simulink model "platoon_project_string_stability3"  (Simulink 8.9)
settings: Solver=FixedStepAuto  StartTime=0.0  StopTime=80  FixedStep=0.02  RelTol=1e-3  EnableMultiTasking=on
model workspace (MAT data in the model file):
  Kd_brake = 1
  Kd_throttle = 500
  Ki_brake = 1
  Ki_throttle = 120
  Kp_brake = 8000
  Kp_throttle = 50
  L = 15
  V0 = 21
  k1 = 0.001
  k2 = -1.004
  q = 0.2
  tau : num (value not decoded)
undefined symbols (not defined in the file): c_aero, delay_brake, F_roll, h, I_e, I_wheel, KB, mass, max_throttle, max_throttle_rate, min_throttle, mu_B, mu_C, mu_D, mu_E, P_po, Rdrive, sigbuilder_block, tau_brake, tau_throttle, throttle_o, tnet_table, w_wheel_o, we_max, we_min, we_o, x_dot_o
libraries: simulink x6
(part 1 of 2)
settings Model: Creator=user  LastModifiedBy=edward
settings SolverCC: AutoInsertRateTranBlk=on
settings DataIOCC: SaveOutput=off  SaveTime=off
settings OptimizationCC: DefaultParameterBehavior=Inlined  InlineInvariantSignals=on  PassReuseOutputArgsAs=Individual arguments  ExpressionDepthLimit=2147483647  StateBitsets=on  DataBitsets=on  ZeroExternalMemoryAtStartup=off  ZeroInternalMemoryAtStartup=off  NoFixptDivByZeroProtection=on  LifeSpan=1
settings DebuggingCC: SolverPrmCheckMsg=warning  ParameterTunabilityLossMsg=error  FcnCallInpInsideContextMsg=error
settings HardwareCC: ProdIntDivRoundTo=Floor  ProdEndianess=LittleEndian  ProdHWDeviceType=Generic->Custom
settings SFSimCC: MATLABDynamicMemAlloc=off
settings RTWCC: SystemTargetFile=ert.tlc  TLCOptions=-p0  GenCodeOnly=on  TemplateMakefile=ert_default_tmf  Description=Embedded Coder  GenerateReport=on  RTWVerbose=off  IncludeHyperlinkInReport=on  LaunchReport=on  GenerateTraceInfo=on  GenerateTraceReport=on  GenerateTraceReportSl=on  GenerateTraceReportSf=on  GenerateTraceReportEml=on
settings CodeAppCC: ForceParamTrailComments=on  IgnoreCustomStorageClasses=off  OperatorAnnotations=on  SimulinkDataObjDesc=on  SFDataObjDesc=on  MATLABFcnDesc=on  CustomSymbolStrGlobalVar=rt$N$M  CustomSymbolStrType=$N$M  CustomSymbolStrFcn=$N$M$F  CustomSymbolStrMacro=$N$M  InsertBlockDesc=on  MATLABSourceComments=on
settings ERTTargetCC: CodeReplacementLibrary=ISO_C  GenerateSampleERTMain=on  IncludeMdlTerminateFcn=off  SuppressErrorStatus=on  SupportAbsoluteTime=off  SupportNonFinite=off  SupportComplex=off  PurelyIntegerCode=on  InlinedParameterPlacement=NonHierarchical  RootIOFormat=Structure reference  ERTCustomFileTemplate=example_file_process.tlc

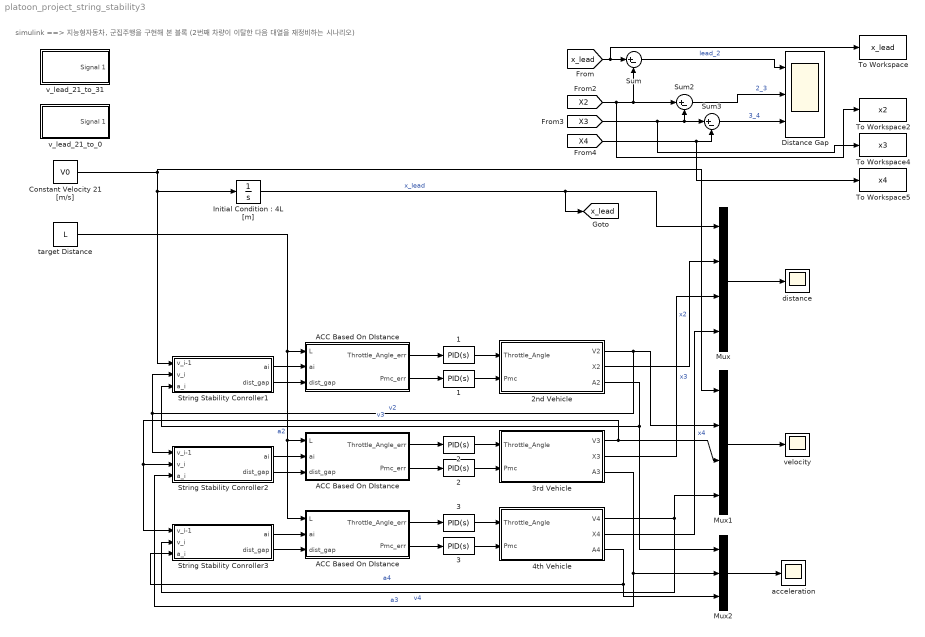
== system platoon_project_string_stability3 ==
  note: simulink ==> 지능형자동차, 군집주행을 구현해 본 블록 (2번째 차량이 이탈한 다음 대열을 재정비하는 시나리오)
  "               ACC Based On DIstance            " : MATLAB Function  TreatAsAtomicUnit=on
  "               ACC Based On DIstance             " : MATLAB Function  TreatAsAtomicUnit=on
  "               ACC Based On DIstance              " : MATLAB Function  TreatAsAtomicUnit=on
  "  1" : simulink/Continuous/PID Controller  Controller=PID  TimeDomain=Continuous-time  SampleTime=-1  IntegratorMethod=Forward Euler  FilterMethod=Forward Euler  Form=Parallel  UseFilter=on  ControllerParametersSource=internal  P=Kp_brake  I=Ki_brake  D=Kd_brake  N=100  InitialConditionSource=internal  InitialConditionForIntegrator=0  InitialConditionForFilter=0  ExternalReset=none  LimitOutput=off  UpperSaturationLimit=inf  LowerSaturationLimit=-inf  LinearizeAsGain=on  AntiWindupMode=none  Kb=1  TrackingMode=off  Kt=1  PParamMin=[]  PParamMax=[]  IParamMin=[]  IParamMax=[]  DParamMin=[]  DParamMax=[]  NParamMin=[]  NParamMax=[]  KbParamMin=[]  KbParamMax=[]  KtParamMin=[]  KtParamMax=[]  POutMin=[]  POutMax=[]  IOutMin=[]  IOutMax=[]  DOutMin=[]  DOutMax=[]  NOutMin=[]  NOutMax=[]  KbOutMin=[]  KbOutMax=[]  KtOutMin=[]  KtOutMax=[]  IntegratorOutMin=[]  IntegratorOutMax=[]  FilterOutMin=[]  FilterOutMax=[]  SumOutMin=[]  SumOutMax=[]  SumI1OutMin=[]  SumI1OutMax=[]  SumI2OutMin=[]  SumI2OutMax=[]  SumI3OutMin=[]  SumI3OutMax=[]  SumDOutMin=[]  SumDOutMax=[]  SaturationOutMin=[]  SaturationOutMax=[]  IntegratorContinuousStateAttributes=''  IntegratorStateMustResolveToSignalObject=off  IntegratorRTWStateStorageClass=Auto  FilterContinuousStateAttributes=''  FilterStateMustResolveToSignalObject=off  FilterRTWStateStorageClass=Auto  DifferentiatorICPrevScaledInput=0  DifferentiatorOutMin=[]  DifferentiatorOutMax=[]  InitialConditionSetting=State (most efficient)
  "  2" : simulink/Continuous/PID Controller  Controller=PID  TimeDomain=Continuous-time  SampleTime=-1  IntegratorMethod=Forward Euler  FilterMethod=Forward Euler  Form=Parallel  UseFilter=on  ControllerParametersSource=internal  P=Kp_brake  I=Ki_brake  D=Kd_brake  N=100  InitialConditionSource=internal  InitialConditionForIntegrator=0  InitialConditionForFilter=0  ExternalReset=none  LimitOutput=off  UpperSaturationLimit=inf  LowerSaturationLimit=-inf  LinearizeAsGain=on  AntiWindupMode=none  Kb=1  TrackingMode=off  Kt=1  PParamMin=[]  PParamMax=[]  IParamMin=[]  IParamMax=[]  DParamMin=[]  DParamMax=[]  NParamMin=[]  NParamMax=[]  KbParamMin=[]  KbParamMax=[]  KtParamMin=[]  KtParamMax=[]  POutMin=[]  POutMax=[]  IOutMin=[]  IOutMax=[]  DOutMin=[]  DOutMax=[]  NOutMin=[]  NOutMax=[]  KbOutMin=[]  KbOutMax=[]  KtOutMin=[]  KtOutMax=[]  IntegratorOutMin=[]  IntegratorOutMax=[]  FilterOutMin=[]  FilterOutMax=[]  SumOutMin=[]  SumOutMax=[]  SumI1OutMin=[]  SumI1OutMax=[]  SumI2OutMin=[]  SumI2OutMax=[]  SumI3OutMin=[]  SumI3OutMax=[]  SumDOutMin=[]  SumDOutMax=[]  SaturationOutMin=[]  SaturationOutMax=[]  IntegratorContinuousStateAttributes=''  IntegratorStateMustResolveToSignalObject=off  IntegratorRTWStateStorageClass=Auto  FilterContinuousStateAttributes=''  FilterStateMustResolveToSignalObject=off  FilterRTWStateStorageClass=Auto  DifferentiatorICPrevScaledInput=0  DifferentiatorOutMin=[]  DifferentiatorOutMax=[]  InitialConditionSetting=State (most efficient)
  "  3" : simulink/Continuous/PID Controller  Controller=PID  TimeDomain=Continuous-time  SampleTime=-1  IntegratorMethod=Forward Euler  FilterMethod=Forward Euler  Form=Parallel  UseFilter=on  ControllerParametersSource=internal  P=Kp_brake  I=Ki_brake  D=Kd_brake  N=100  InitialConditionSource=internal  InitialConditionForIntegrator=0  InitialConditionForFilter=0  ExternalReset=none  LimitOutput=off  UpperSaturationLimit=inf  LowerSaturationLimit=-inf  LinearizeAsGain=on  AntiWindupMode=none  Kb=1  TrackingMode=off  Kt=1  PParamMin=[]  PParamMax=[]  IParamMin=[]  IParamMax=[]  DParamMin=[]  DParamMax=[]  NParamMin=[]  NParamMax=[]  KbParamMin=[]  KbParamMax=[]  KtParamMin=[]  KtParamMax=[]  POutMin=[]  POutMax=[]  IOutMin=[]  IOutMax=[]  DOutMin=[]  DOutMax=[]  NOutMin=[]  NOutMax=[]  KbOutMin=[]  KbOutMax=[]  KtOutMin=[]  KtOutMax=[]  IntegratorOutMin=[]  IntegratorOutMax=[]  FilterOutMin=[]  FilterOutMax=[]  SumOutMin=[]  SumOutMax=[]  SumI1OutMin=[]  SumI1OutMax=[]  SumI2OutMin=[]  SumI2OutMax=[]  SumI3OutMin=[]  SumI3OutMax=[]  SumDOutMin=[]  SumDOutMax=[]  SaturationOutMin=[]  SaturationOutMax=[]  IntegratorContinuousStateAttributes=''  IntegratorStateMustResolveToSignalObject=off  IntegratorRTWStateStorageClass=Auto  FilterContinuousStateAttributes=''  FilterStateMustResolveToSignalObject=off  FilterRTWStateStorageClass=Auto  DifferentiatorICPrevScaledInput=0  DifferentiatorOutMin=[]  DifferentiatorOutMax=[]  InitialConditionSetting=State (most efficient)
  " 1" : simulink/Continuous/PID Controller  Controller=PID  TimeDomain=Continuous-time  SampleTime=-1  IntegratorMethod=Forward Euler  FilterMethod=Forward Euler  Form=Parallel  UseFilter=on  ControllerParametersSource=internal  P=Kp_throttle  I=Ki_throttle  D=Kd_throttle  N=100  InitialConditionSource=internal  InitialConditionForIntegrator=0  InitialConditionForFilter=0  ExternalReset=none  LimitOutput=off  UpperSaturationLimit=inf  LowerSaturationLimit=-inf  LinearizeAsGain=on  AntiWindupMode=none  Kb=1  TrackingMode=off  Kt=1  PParamMin=[]  PParamMax=[]  IParamMin=[]  IParamMax=[]  DParamMin=[]  DParamMax=[]  NParamMin=[]  NParamMax=[]  KbParamMin=[]  KbParamMax=[]  KtParamMin=[]  KtParamMax=[]  POutMin=[]  POutMax=[]  IOutMin=[]  IOutMax=[]  DOutMin=[]  DOutMax=[]  NOutMin=[]  NOutMax=[]  KbOutMin=[]  KbOutMax=[]  KtOutMin=[]  KtOutMax=[]  IntegratorOutMin=[]  IntegratorOutMax=[]  FilterOutMin=[]  FilterOutMax=[]  SumOutMin=[]  SumOutMax=[]  SumI1OutMin=[]  SumI1OutMax=[]  SumI2OutMin=[]  SumI2OutMax=[]  SumI3OutMin=[]  SumI3OutMax=[]  SumDOutMin=[]  SumDOutMax=[]  SaturationOutMin=[]  SaturationOutMax=[]  IntegratorContinuousStateAttributes=''  IntegratorStateMustResolveToSignalObject=off  IntegratorRTWStateStorageClass=Auto  FilterContinuousStateAttributes=''  FilterStateMustResolveToSignalObject=off  FilterRTWStateStorageClass=Auto  DifferentiatorICPrevScaledInput=0  DifferentiatorOutMin=[]  DifferentiatorOutMax=[]  InitialConditionSetting=State (most efficient)
  " 2" : simulink/Continuous/PID Controller  Controller=PID  TimeDomain=Continuous-time  SampleTime=-1  IntegratorMethod=Forward Euler  FilterMethod=Forward Euler  Form=Parallel  UseFilter=on  ControllerParametersSource=internal  P=Kp_throttle  I=Ki_throttle  D=Kd_throttle  N=100  InitialConditionSource=internal  InitialConditionForIntegrator=0  InitialConditionForFilter=0  ExternalReset=none  LimitOutput=off  UpperSaturationLimit=inf  LowerSaturationLimit=-inf  LinearizeAsGain=on  AntiWindupMode=none  Kb=1  TrackingMode=off  Kt=1  PParamMin=[]  PParamMax=[]  IParamMin=[]  IParamMax=[]  DParamMin=[]  DParamMax=[]  NParamMin=[]  NParamMax=[]  KbParamMin=[]  KbParamMax=[]  KtParamMin=[]  KtParamMax=[]  POutMin=[]  POutMax=[]  IOutMin=[]  IOutMax=[]  DOutMin=[]  DOutMax=[]  NOutMin=[]  NOutMax=[]  KbOutMin=[]  KbOutMax=[]  KtOutMin=[]  KtOutMax=[]  IntegratorOutMin=[]  IntegratorOutMax=[]  FilterOutMin=[]  FilterOutMax=[]  SumOutMin=[]  SumOutMax=[]  SumI1OutMin=[]  SumI1OutMax=[]  SumI2OutMin=[]  SumI2OutMax=[]  SumI3OutMin=[]  SumI3OutMax=[]  SumDOutMin=[]  SumDOutMax=[]  SaturationOutMin=[]  SaturationOutMax=[]  IntegratorContinuousStateAttributes=''  IntegratorStateMustResolveToSignalObject=off  IntegratorRTWStateStorageClass=Auto  FilterContinuousStateAttributes=''  FilterStateMustResolveToSignalObject=off  FilterRTWStateStorageClass=Auto  DifferentiatorICPrevScaledInput=0  DifferentiatorOutMin=[]  DifferentiatorOutMax=[]  InitialConditionSetting=State (most efficient)
  " 3" : simulink/Continuous/PID Controller  Controller=PID  TimeDomain=Continuous-time  SampleTime=-1  IntegratorMethod=Forward Euler  FilterMethod=Forward Euler  Form=Parallel  UseFilter=on  ControllerParametersSource=internal  P=Kp_throttle  I=Ki_throttle  D=Kd_throttle  N=100  InitialConditionSource=internal  InitialConditionForIntegrator=0  InitialConditionForFilter=0  ExternalReset=none  LimitOutput=off  UpperSaturationLimit=inf  LowerSaturationLimit=-inf  LinearizeAsGain=on  AntiWindupMode=none  Kb=1  TrackingMode=off  Kt=1  PParamMin=[]  PParamMax=[]  IParamMin=[]  IParamMax=[]  DParamMin=[]  DParamMax=[]  NParamMin=[]  NParamMax=[]  KbParamMin=[]  KbParamMax=[]  KtParamMin=[]  KtParamMax=[]  POutMin=[]  POutMax=[]  IOutMin=[]  IOutMax=[]  DOutMin=[]  DOutMax=[]  NOutMin=[]  NOutMax=[]  KbOutMin=[]  KbOutMax=[]  KtOutMin=[]  KtOutMax=[]  IntegratorOutMin=[]  IntegratorOutMax=[]  FilterOutMin=[]  FilterOutMax=[]  SumOutMin=[]  SumOutMax=[]  SumI1OutMin=[]  SumI1OutMax=[]  SumI2OutMin=[]  SumI2OutMax=[]  SumI3OutMin=[]  SumI3OutMax=[]  SumDOutMin=[]  SumDOutMax=[]  SaturationOutMin=[]  SaturationOutMax=[]  IntegratorContinuousStateAttributes=''  IntegratorStateMustResolveToSignalObject=off  IntegratorRTWStateStorageClass=Auto  FilterContinuousStateAttributes=''  FilterStateMustResolveToSignalObject=off  FilterRTWStateStorageClass=Auto  DifferentiatorICPrevScaledInput=0  DifferentiatorOutMin=[]  DifferentiatorOutMax=[]  InitialConditionSetting=State (most efficient)
  2nd Vehicle : Subsystem
  3rd Vehicle : Subsystem
  4th Vehicle : Subsystem
  Constant Velocity 21 [m/s] : Constant  Value=V0
  Distance Gap : Scope  NumInputPorts=3
  "Initial Condition : 4L [m]" : Integrator  InitialCondition=4*L
  Mux : Mux
  Mux1 : Mux
  Mux2 : Mux  Inputs=3
  String Stability Conroller1 : Subsystem
  String Stability Conroller2 : Subsystem
  String Stability Conroller3 : Subsystem
  Sum : Sum  Inputs=|+-
  Sum2 : Sum  Inputs=|+-
  Sum3 : Sum  Inputs=|+-
  To Workspace : ToWorkspace  VariableName=x_lead  SampleTime=-1
  To Workspace2 : ToWorkspace  VariableName=x2  SampleTime=-1
  To Workspace4 : ToWorkspace  VariableName=x3  SampleTime=-1
  To Workspace5 : ToWorkspace  VariableName=x4  SampleTime=-1
  acceleration : Scope
  distance : Scope
  target Distance : Constant  Value=L
  v_lead_21_to_0 : Subsystem  Tag=STV Subsys  LoadFcn=sigbuilder_block('load');  StartFcn=sigbuilder_block('start');  StopFcn=sigbuilder_block('stop');  ClipboardFcn=sigbuilder_block('clipboard');  mask(Sigbuilder block){tuvar=[0:10]}
      mask help: Simulink:masks:SigbuilderBlock_MD
      mask init:
      | if ~strcmp(get_param(bdroot(gcbh),'SimulationStatus'),'stopped') tuvar = sigbuilder_block('maskInit'); end
      settings: CopyFcn=sigbuilder_block('copy');  DeleteFcn=sigbuilder_block('delete');  ModelCloseFcn=sigbuilder_block('modelClose');  PreSaveFcn=sigbuilder_block('preSave');  PauseFcn=sigbuilder_block('pause');  ContinueFcn=sigbuilder_block('continue');  NameChangeFcn=sigbuilder_block('namechange');  OpenFcn=sigbuilder_block('open',[434.4 168 550.8 400.2 ]);  CloseFcn=sigbuilder_block('close');
      mask Display: plot(0, 0, 100, 100,[2, 2, 32, 32, 2], [68, 8, 8, 68, 68],[32, 2], [38, 38], [32, 19, 2],[53, 60, 44], [32, 17, 17, 2],[16, 16, 31, 31]);txt = getActiveGroup(gcbh);text(2, 100, txt,'verticalAlignment', 'top');
  v_lead_21_to_31 : Subsystem  Tag=STV Subsys  LoadFcn=sigbuilder_block('load');  StartFcn=sigbuilder_block('start');  StopFcn=sigbuilder_block('stop');  ClipboardFcn=sigbuilder_block('clipboard');  mask(Sigbuilder block){tuvar=[0:10]}
      mask help: Simulink:masks:SigbuilderBlock_MD
      mask init:
      | if ~strcmp(get_param(bdroot(gcbh),'SimulationStatus'),'stopped') tuvar = sigbuilder_block('maskInit'); end
      settings: CopyFcn=sigbuilder_block('copy');  DeleteFcn=sigbuilder_block('delete');  ModelCloseFcn=sigbuilder_block('modelClose');  PreSaveFcn=sigbuilder_block('preSave');  PauseFcn=sigbuilder_block('pause');  ContinueFcn=sigbuilder_block('continue');  NameChangeFcn=sigbuilder_block('namechange');  OpenFcn=sigbuilder_block('open',[434.4 168 550.8 400.2 ]);  CloseFcn=sigbuilder_block('close');
      mask Display: plot(0, 0, 100, 100,[2, 2, 32, 32, 2], [68, 8, 8, 68, 68],[32, 2], [38, 38], [32, 19, 2],[53, 60, 44], [32, 17, 17, 2],[16, 16, 31, 31]);txt = getActiveGroup(gcbh);text(2, 100, txt,'verticalAlignment', 'top');
  velocity : Scope
  tag scope: x_lead=global
  wires:
  "Initial Condition : 4L [m]"/1 -> Mux/1, [x_lead]  "x_lead"
  " 1"/1 -> 2nd Vehicle/1(Throttle_Angle)
  "  1"/1 -> 2nd Vehicle/2(Pmc)
  Mux/1 -> distance/1
  String Stability Conroller1/1(ai) -> "               ACC Based On DIstance            "/2(ai)
  "               ACC Based On DIstance            "/2(Pmc_err) -> "  1"/1
  "               ACC Based On DIstance            "/1(Throttle_Angle_err) -> " 1"/1
  2nd Vehicle/1(V2) -> Mux1/2, String Stability Conroller2/1(v_i-1), String Stability Conroller1/2(v_i)  "v2"
  2nd Vehicle/3(A2) -> Mux2/1, String Stability Conroller1/3(a_i)  "a2"
  2nd Vehicle/2(X2) -> Mux/2  "x2"
  Mux2/1 -> acceleration/1
  "               ACC Based On DIstance              "/1(Throttle_Angle_err) -> " 2"/1
  "               ACC Based On DIstance              "/2(Pmc_err) -> "  2"/1
  String Stability Conroller2/1(ai) -> "               ACC Based On DIstance              "/2(ai)
  String Stability Conroller3/1(ai) -> "               ACC Based On DIstance             "/2(ai)
  "               ACC Based On DIstance             "/2(Pmc_err) -> "  3"/1
  "               ACC Based On DIstance             "/1(Throttle_Angle_err) -> " 3"/1
  " 2"/1 -> 3rd Vehicle/1(Throttle_Angle)
  "  2"/1 -> 3rd Vehicle/2(Pmc)
  " 3"/1 -> 4th Vehicle/1(Throttle_Angle)
  "  3"/1 -> 4th Vehicle/2(Pmc)
  3rd Vehicle/1(V3) -> Mux1/3, String Stability Conroller3/1(v_i-1), String Stability Conroller2/2(v_i)  "v3"
  3rd Vehicle/3(A3) -> Mux2/2, String Stability Conroller2/3(a_i)  "a3"
  3rd Vehicle/2(X3) -> Mux/3  "x3"
  4th Vehicle/2(X4) -> Mux/4  "x4"
  4th Vehicle/1(V4) -> Mux1/4, String Stability Conroller3/2(v_i)  "v4"
  4th Vehicle/3(A4) -> Mux2/3, String Stability Conroller3/3(a_i)  "a4"
  Constant Velocity 21 [m/s]/1 -> Mux1/1, String Stability Conroller1/1(v_i-1), "Initial Condition : 4L [m]"/1
  [x_lead] -> To Workspace/1, Sum/1
  [X3] -> To Workspace4/1, Sum3/1, Sum2/2
  [X4] -> To Workspace5/1, Sum3/2
  Sum/1 -> Distance Gap/1  "lead_2"
  Sum2/1 -> Distance Gap/2  "2_3"
  Sum3/1 -> Distance Gap/3  "3_4"
  String Stability Conroller1/2(dist_gap) -> "               ACC Based On DIstance            "/3(dist_gap)
  String Stability Conroller2/2(dist_gap) -> "               ACC Based On DIstance              "/3(dist_gap)
  String Stability Conroller3/2(dist_gap) -> "               ACC Based On DIstance             "/3(dist_gap)
  [X2] -> To Workspace2/1, Sum/2, Sum2/1
  target Distance/1 -> "               ACC Based On DIstance             "/1(L), "               ACC Based On DIstance              "/1(L), "               ACC Based On DIstance            "/1(L)
  Mux1/1 -> velocity/1

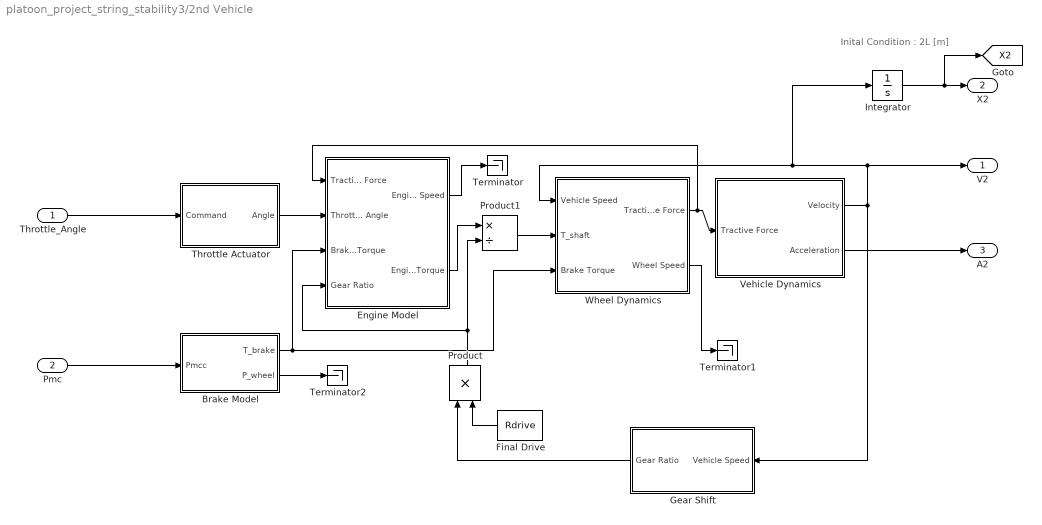
== system platoon_project_string_stability3/2nd Vehicle ==
  note: Inital Condition : 2L [m]
  Throttle_Angle : Inport
  Pmc : Inport  Port=2
  Brake Model : Subsystem
  Engine Model : Subsystem
  Final Drive : Constant  Value=Rdrive
  Gear Shift : Subsystem
  Integrator : Integrator  InitialCondition=2*L
  Product : Product  Inputs=**  SaturateOnIntegerOverflow=on  RndMeth=Zero  InputSameDT=on  OutDataTypeStr=Inherit: Same as first input
  Product1 : Product  Inputs=*/  SaturateOnIntegerOverflow=on  RndMeth=Zero  InputSameDT=on  OutDataTypeStr=Inherit: Same as first input
  Terminator : Terminator
  Terminator1 : Terminator
  Terminator2 : Terminator
  Throttle Actuator : Subsystem
  Vehicle Dynamics : Subsystem
  Wheel Dynamics : Subsystem
  V2 : Outport
  X2 : Outport  Port=2
  A2 : Outport  Port=3
  tag scope: X2=global
  wires:
  Integrator/1 -> [X2], X2/1
  Vehicle Dynamics/2(Acceleration) -> A2/1
  Brake Model/2(P_wheel) -> Terminator2/1
  Wheel Dynamics/2(Wheel Speed) -> Terminator1/1
  Engine Model/1(Engine Speed) -> Terminator/1
  Product1/1 -> Wheel Dynamics/2(T_shaft)
  Engine Model/2(Engine Torque) -> Product1/1
  Brake Model/1(T_brake) -> Engine Model/3(Brake Torque), Wheel Dynamics/3(Brake Torque)
  Product/1 -> Product1/2, Engine Model/4(Gear Ratio)
  Final Drive/1 -> Product/2
  Gear Shift/1(Gear Ratio) -> Product/1
  Wheel Dynamics/1(Tractive Force) -> Vehicle Dynamics/1(Tractive Force), Engine Model/1(Tractive Force)
  Throttle Actuator/1(Angle) -> Engine Model/2(Throttle Angle)
  Throttle_Angle/1 -> Throttle Actuator/1(Command)
  Pmc/1 -> Brake Model/1(Pmcc)
  Vehicle Dynamics/1(Velocity) -> Wheel Dynamics/1(Vehicle Speed), Integrator/1, V2/1, Gear Shift/1(Vehicle Speed)

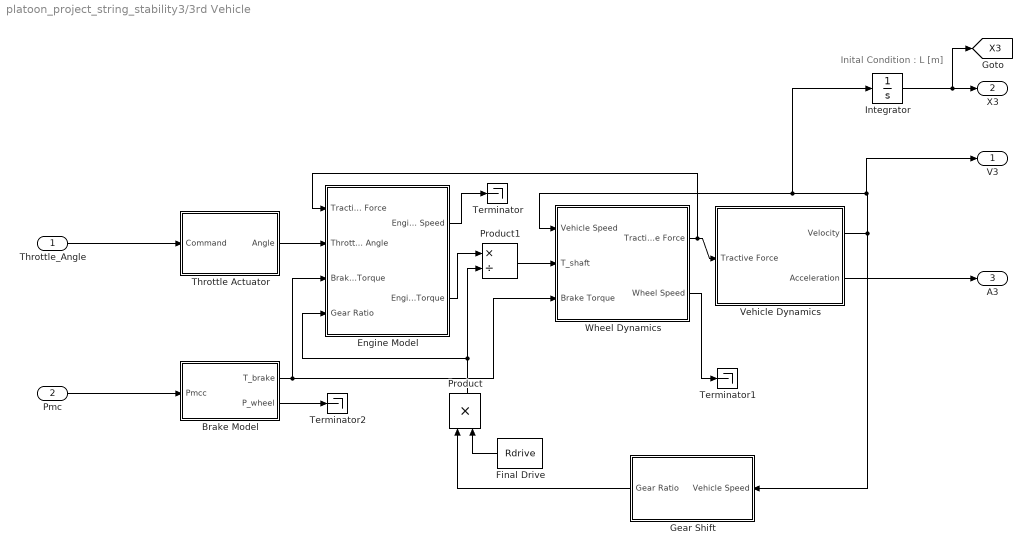
== system platoon_project_string_stability3/3rd Vehicle ==
  note: Inital Condition : L [m]
  Throttle_Angle : Inport
  Pmc : Inport  Port=2
  Brake Model : Subsystem
  Engine Model : Subsystem
  Final Drive : Constant  Value=Rdrive
  Gear Shift : Subsystem
  Integrator : Integrator  InitialCondition=L
  Product : Product  Inputs=**  SaturateOnIntegerOverflow=on  RndMeth=Zero  InputSameDT=on  OutDataTypeStr=Inherit: Same as first input
  Product1 : Product  Inputs=*/  SaturateOnIntegerOverflow=on  RndMeth=Zero  InputSameDT=on  OutDataTypeStr=Inherit: Same as first input
  Terminator : Terminator
  Terminator1 : Terminator
  Terminator2 : Terminator
  Throttle Actuator : Subsystem
  Vehicle Dynamics : Subsystem
  Wheel Dynamics : Subsystem
  V3 : Outport
  X3 : Outport  Port=2
  A3 : Outport  Port=3
  tag scope: X3=global
  wires:
  Pmc/1 -> Brake Model/1(Pmcc)
  Throttle_Angle/1 -> Throttle Actuator/1(Command)
  Throttle Actuator/1(Angle) -> Engine Model/2(Throttle Angle)
  Wheel Dynamics/1(Tractive Force) -> Engine Model/1(Tractive Force), Vehicle Dynamics/1(Tractive Force)
  Gear Shift/1(Gear Ratio) -> Product/1
  Final Drive/1 -> Product/2
  Product/1 -> Engine Model/4(Gear Ratio), Product1/2
  Brake Model/1(T_brake) -> Wheel Dynamics/3(Brake Torque), Engine Model/3(Brake Torque)
  Engine Model/2(Engine Torque) -> Product1/1
  Product1/1 -> Wheel Dynamics/2(T_shaft)
  Engine Model/1(Engine Speed) -> Terminator/1
  Wheel Dynamics/2(Wheel Speed) -> Terminator1/1
  Brake Model/2(P_wheel) -> Terminator2/1
  Vehicle Dynamics/2(Acceleration) -> A3/1
  Vehicle Dynamics/1(Velocity) -> Gear Shift/1(Vehicle Speed), V3/1, Integrator/1, Wheel Dynamics/1(Vehicle Speed)
  Integrator/1 -> [X3], X3/1

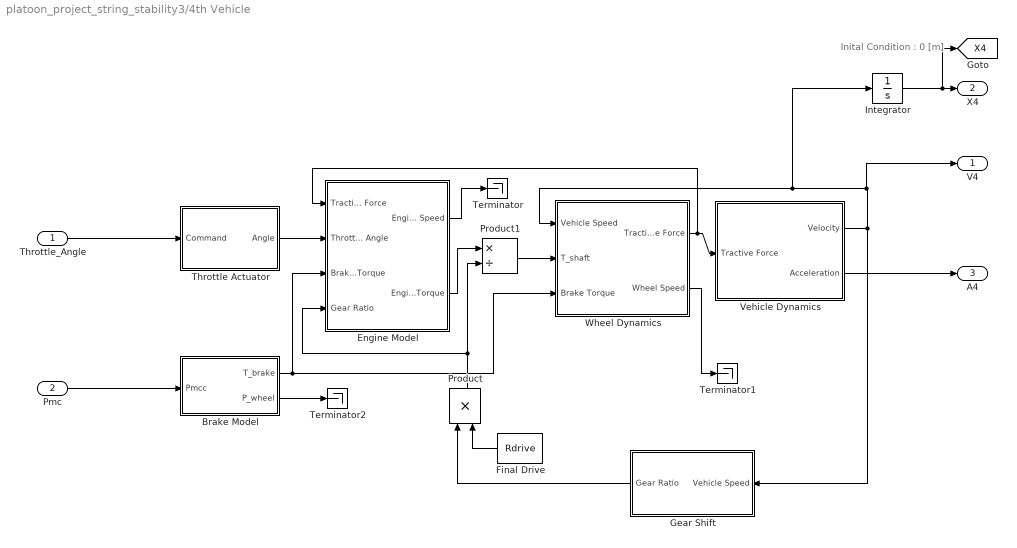
== system platoon_project_string_stability3/4th Vehicle ==
  note: Inital Condition : 0 [m]
  Throttle_Angle : Inport
  Pmc : Inport  Port=2
  Brake Model : Subsystem
  Engine Model : Subsystem
  Final Drive : Constant  Value=Rdrive
  Gear Shift : Subsystem
  Integrator : Integrator
  Product : Product  Inputs=**  SaturateOnIntegerOverflow=on  RndMeth=Zero  InputSameDT=on  OutDataTypeStr=Inherit: Same as first input
  Product1 : Product  Inputs=*/  SaturateOnIntegerOverflow=on  RndMeth=Zero  InputSameDT=on  OutDataTypeStr=Inherit: Same as first input
  Terminator : Terminator
  Terminator1 : Terminator
  Terminator2 : Terminator
  Throttle Actuator : Subsystem
  Vehicle Dynamics : Subsystem
  Wheel Dynamics : Subsystem
  V4 : Outport
  X4 : Outport  Port=2
  A4 : Outport  Port=3
  tag scope: X4=global
  wires:
  Integrator/1 -> [X4], X4/1
  Vehicle Dynamics/2(Acceleration) -> A4/1
  Brake Model/2(P_wheel) -> Terminator2/1
  Wheel Dynamics/2(Wheel Speed) -> Terminator1/1
  Engine Model/1(Engine Speed) -> Terminator/1
  Product1/1 -> Wheel Dynamics/2(T_shaft)
  Engine Model/2(Engine Torque) -> Product1/1
  Brake Model/1(T_brake) -> Engine Model/3(Brake Torque), Wheel Dynamics/3(Brake Torque)
  Product/1 -> Product1/2, Engine Model/4(Gear Ratio)
  Final Drive/1 -> Product/2
  Gear Shift/1(Gear Ratio) -> Product/1
  Wheel Dynamics/1(Tractive Force) -> Vehicle Dynamics/1(Tractive Force), Engine Model/1(Tractive Force)
  Throttle Actuator/1(Angle) -> Engine Model/2(Throttle Angle)
  Throttle_Angle/1 -> Throttle Actuator/1(Command)
  Pmc/1 -> Brake Model/1(Pmcc)
  Vehicle Dynamics/1(Velocity) -> V4/1, Wheel Dynamics/1(Vehicle Speed), Integrator/1, Gear Shift/1(Vehicle Speed)

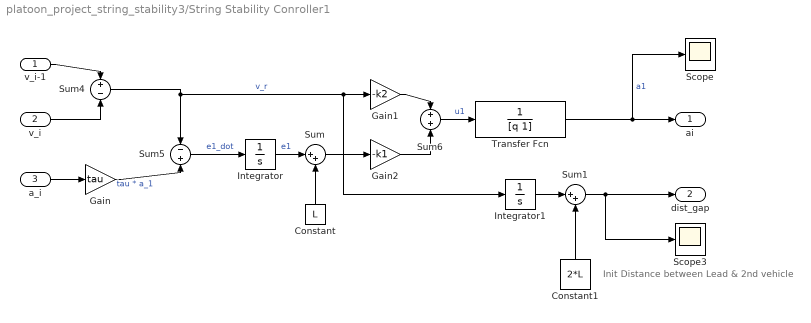
== system platoon_project_string_stability3/String Stability Conroller1 ==
  note: Init Distance between Lead & 2nd vehicle
  v_i-1 : Inport
  v_i : Inport  Port=2
  a_i : Inport  Port=3
  Constant : Constant  Value=L
  Constant1 : Constant  Value=2*L
  Gain : Gain  Gain=tau
  Gain1 : Gain  Gain=-k2
  Gain2 : Gain  Gain=-k1
  Integrator : Integrator
  Integrator1 : Integrator
  Scope : Scope
  Scope3 : Scope
  Sum : Sum  Inputs=|++
  Sum1 : Sum  Inputs=|++
  Sum4 : Sum  Inputs=+|-
  Sum5 : Sum  Inputs=-|+
  Sum6 : Sum  Inputs=+|+
  Transfer Fcn : TransferFcn  Denominator=[q 1]
  ai : Outport
  dist_gap : Outport  Port=2
  wires:
  v_i-1/1 -> Sum4/1
  v_i/1 -> Sum4/2
  a_i/1 -> Gain/1
  Sum6/1 -> Transfer Fcn/1  "u1"
  Gain/1 -> Sum5/2  "tau * a_1"
  Sum5/1 -> Integrator/1  "e1_dot"
  Gain2/1 -> Sum6/2
  Gain1/1 -> Sum6/1
  Transfer Fcn/1 -> Scope/1, ai/1  "a1"
  Constant/1 -> Sum/2
  Sum/1 -> Gain2/1
  Integrator/1 -> Sum/1  "e1"
  Sum4/1 -> Integrator1/1, Gain1/1, Sum5/1  "v_r"
  Integrator1/1 -> Sum1/1
  Sum1/1 -> dist_gap/1, Scope3/1
  Constant1/1 -> Sum1/2

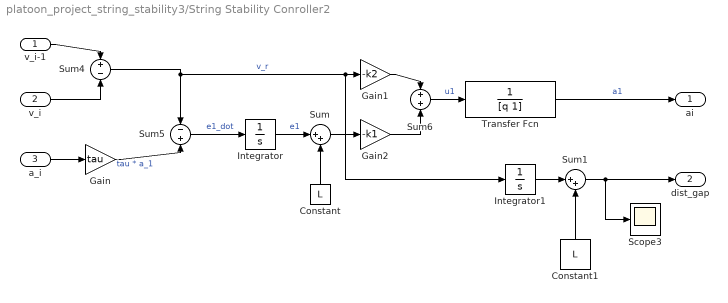
== system platoon_project_string_stability3/String Stability Conroller2 ==
  v_i-1 : Inport
  v_i : Inport  Port=2
  a_i : Inport  Port=3
  Constant : Constant  Value=L
  Constant1 : Constant  Value=L
  Gain : Gain  Gain=tau
  Gain1 : Gain  Gain=-k2
  Gain2 : Gain  Gain=-k1
  Integrator : Integrator
  Integrator1 : Integrator
  Scope3 : Scope
  Sum : Sum  Inputs=|++
  Sum1 : Sum  Inputs=|++
  Sum4 : Sum  Inputs=+|-
  Sum5 : Sum  Inputs=-|+
  Sum6 : Sum  Inputs=+|+
  Transfer Fcn : TransferFcn  Denominator=[q 1]
  ai : Outport
  dist_gap : Outport  Port=2
  wires:
  Gain1/1 -> Sum6/1
  Gain2/1 -> Sum6/2
  Sum5/1 -> Integrator/1  "e1_dot"
  Gain/1 -> Sum5/2  "tau * a_1"
  Sum6/1 -> Transfer Fcn/1  "u1"
  Transfer Fcn/1 -> ai/1  "a1"
  a_i/1 -> Gain/1
  v_i/1 -> Sum4/2
  v_i-1/1 -> Sum4/1
  Constant/1 -> Sum/2
  Sum/1 -> Gain2/1
  Integrator/1 -> Sum/1  "e1"
  Sum4/1 -> Sum5/1, Integrator1/1, Gain1/1  "v_r"
  Integrator1/1 -> Sum1/1
  Sum1/1 -> dist_gap/1, Scope3/1
  Constant1/1 -> Sum1/2

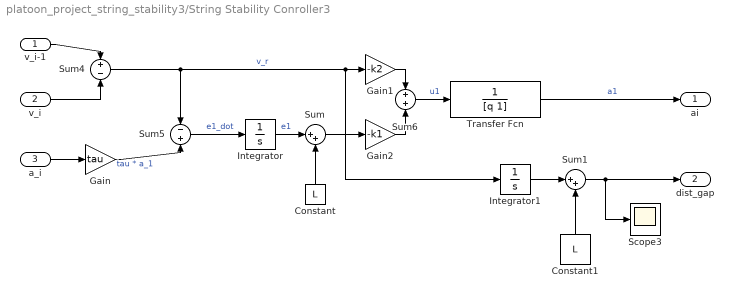
== system platoon_project_string_stability3/String Stability Conroller3 ==
  v_i-1 : Inport
  v_i : Inport  Port=2
  a_i : Inport  Port=3
  Constant : Constant  Value=L
  Constant1 : Constant  Value=L
  Gain : Gain  Gain=tau
  Gain1 : Gain  Gain=-k2
  Gain2 : Gain  Gain=-k1
  Integrator : Integrator
  Integrator1 : Integrator
  Scope3 : Scope
  Sum : Sum  Inputs=|++
  Sum1 : Sum  Inputs=|++
  Sum4 : Sum  Inputs=+|-
  Sum5 : Sum  Inputs=-|+
  Sum6 : Sum  Inputs=+|+
  Transfer Fcn : TransferFcn  Denominator=[q 1]
  ai : Outport
  dist_gap : Outport  Port=2
  wires:
  v_i-1/1 -> Sum4/1
  v_i/1 -> Sum4/2
  a_i/1 -> Gain/1
  Transfer Fcn/1 -> ai/1  "a1"
  Sum6/1 -> Transfer Fcn/1  "u1"
  Gain/1 -> Sum5/2  "tau * a_1"
  Sum5/1 -> Integrator/1  "e1_dot"
  Gain2/1 -> Sum6/2
  Gain1/1 -> Sum6/1
  Constant/1 -> Sum/2
  Sum/1 -> Gain2/1
  Integrator/1 -> Sum/1  "e1"
  Sum4/1 -> Sum5/1, Integrator1/1, Gain1/1  "v_r"
  Integrator1/1 -> Sum1/1
  Sum1/1 -> dist_gap/1, Scope3/1
  Constant1/1 -> Sum1/2

== system platoon_project_string_stability3/v_lead_21_to_0 ==
  Demux : Demux  Tag=STV Demux  Outputs=1
  FromWs : FromWorkspace  Tag=STV FromWs  VariableName=tuvar  SampleTime=0  SigBuilderData=DataTag1  VnvData=DataTag2
      SigBuilderData=|
      | common.afterFinalStr = 'Extrapolate'
      | common.sampleTime = 0
      | dataSet.timeRange = [0 20]
      | dataSet.name = 'Senario 2'
      | sbobj.Groups.Name = 'Senario 2'
      | sbobj.Groups.Signals.Name = 'Signal 1'
      | sbobj.Groups.Signals.XData = [0 5 8 20]
      | sbobj.Groups.Signals.YData = [21 21 5 5]
      | sbobj.Groups.TimeRange = [0 20]
  Signal 1 : Outport  Tag=STV Outport
  wires:
  Demux/1 -> Signal 1/1
  FromWs/1 -> Demux/1

== system platoon_project_string_stability3/v_lead_21_to_31 ==
  Demux : Demux  Tag=STV Demux  Outputs=1
  FromWs : FromWorkspace  Tag=STV FromWs  VariableName=tuvar  SampleTime=0  SigBuilderData=DataTag3  VnvData=DataTag4
      SigBuilderData=|
      | common.afterFinalStr = 'Extrapolate'
      | common.sampleTime = 0
      | dataSet.timeRange = [0 20]
      | dataSet.name = 'Senario 1'
      | sbobj.Groups.Name = 'Senario 1'
      | sbobj.Groups.Signals.Name = 'Signal 1'
      | sbobj.Groups.Signals.XData = [0 5 8 20]
      | sbobj.Groups.Signals.YData = [21 21 31 31]
      | sbobj.Groups.TimeRange = [0 20]
  Signal 1 : Outport  Tag=STV Outport
  wires:
  FromWs/1 -> Demux/1
  Demux/1 -> Signal 1/1

== system platoon_project_string_stability3/2nd Vehicle/Brake Model ==
  note: Wheel Pressure가 브레이크 패드에 있는
      | Spring(k)보다 크게 걸렸을 때에만 브레이크가 작동하므로
      | Dead Zone이 발생한다
  note: Wheel pressure
  note: brake는 1차 전달함수의 response를 보인다
  note: Valve를 여닫는 시간에 따라
      | 필연적으로 발생하는 Time Delay
  Pmcc : Inport
  Brake Coefficient : Gain  Gain=KB  SaturateOnIntegerOverflow=on  OutDataTypeStr=Inherit: Same as input  ParamDataTypeStr=Inherit: Same as input
  Brake Dynamics : TransferFcn  Denominator=[tau_brake 1]
  Dead Zone : DeadZone  LowerValue=-P_po  UpperValue=P_po  SaturateOnIntegerOverflow=on
  Pure Time Delay : TransportDelay  DelayTime=delay_brake
  T_brake : Outport
  P_wheel : Outport  Port=2
  wires:
  Brake Coefficient/1 -> T_brake/1
  Dead Zone/1 -> Brake Coefficient/1
  Brake Dynamics/1 -> P_wheel/1, Dead Zone/1  "P_wheel"
  Pmcc/1 -> Pure Time Delay/1
  Pure Time Delay/1 -> Brake Dynamics/1

== system platoon_project_string_stability3/2nd Vehicle/Engine Model ==
  note: engine map이 저장되어있다
      | 2-D Lookup table
      |
      | input : Throttle angle, Engine speed
      | output : Engine torque
  Tractive Force : Inport
  Throttle Angle : Inport  Port=2
  Brake Torque : Inport  Port=3
  Gear Ratio : Inport  Port=4
  1/(I_e+4*I_w*R^2) : Fcn  Expr=u(1)/(I_e+4*I_wheel*u(2)^2)
  Integrator : Integrator  InitialCondition=we_o  LimitOutput=on  UpperSaturationLimit=[we_max]  LowerSaturationLimit=[we_min]
  Mux : Mux  Inputs=2
  Product : Product  SaturateOnIntegerOverflow=on  RndMeth=Zero  InputSameDT=on  OutDataTypeStr=Inherit: Same as first input
  Sum : Sum  Inputs=+|-  SaturateOnIntegerOverflow=on  InputSameDT=on  OutDataTypeStr=Inherit: Same as first input
  Sum1 : Sum  SaturateOnIntegerOverflow=on  InputSameDT=on  OutDataTypeStr=Inherit: Same as first input
  T_net : Lookup2D  RowIndex=alpha_table  ColumnIndex=we_table  Table=tnet_table  SaturateOnIntegerOverflow=on  InputSameDT=on
  wheel radius : Gain  Gain=h  Multiplication=Matrix(K*u)  SaturateOnIntegerOverflow=on  OutDataTypeStr=Inherit: Same as input  ParamDataTypeStr=Inherit: Same as input
  Engine Speed : Outport
  Engine Torque : Outport  Port=2
  wires:
  Throttle Angle/1 -> T_net/1
  Integrator/1 -> Engine Speed/1, T_net/2  "w"
  1/(I_e+4*I_w*R^2)/1 -> Integrator/1  "w_dot"
  Tractive Force/1 -> wheel radius/1
  wheel radius/1 -> Sum1/1
  Brake Torque/1 -> Sum1/2
  Product/1 -> Sum/2
  Sum1/1 -> Product/1
  Gear Ratio/1 -> Product/2, Mux/2
  Sum/1 -> Mux/1
  Mux/1 -> 1/(I_e+4*I_w*R^2)/1
  T_net/1 -> Engine Torque/1, Sum/1

== system platoon_project_string_stability3/2nd Vehicle/Gear Shift ==
  note: [1 1 1]인 [n,1] 행렬과
      | 반환행렬을 곱해서
      | 스칼라값(기어값)을 만든다
  note: 현재 차량 속도 vs 기어변속 속도를 비교한다
      | [0; 1; 1] 같은 [1,n]행렬이 반환된다
  Vehicle Speed : Inport
  Convert m/s to mph : Gain  Gain=3.6/1.6  SaturateOnIntegerOverflow=on  OutDataTypeStr=Inherit: Same as input  ParamDataTypeStr=Inherit: Same as input
  Direct Look-Up of Gear ratio : LookupNDDirect  NumberOfTableDimensions=1  Table=[0.3423,0.6378,1.0,1.4184]
  Get gear-1 : Gain  Gain=ones(1,3)  Multiplication=Matrix(K*u)  SaturateOnIntegerOverflow=on  OutDataTypeStr=Inherit: Same as input  ParamDataTypeStr=Inherit: Same as input
  Relational Operator : RelationalOperator  Operator=>  RndMeth=Nearest  InputSameDT=on
  Shift Speeds : Constant  Value=[15 32 67]
  Gear Ratio : Outport
  wires:
  Shift Speeds/1 -> Relational Operator/2
  Relational Operator/1 -> Get gear-1/1
  Convert m/s to mph/1 -> Relational Operator/1
  Get gear-1/1 -> Direct Look-Up of Gear ratio/1
  Vehicle Speed/1 -> Convert m/s to mph/1
  Direct Look-Up of Gear ratio/1 -> Gear Ratio/1

== system platoon_project_string_stability3/2nd Vehicle/Throttle Actuator ==
  Command : Inport
  Integrator : Integrator  InitialCondition=throttle_o  LimitOutput=on  UpperSaturationLimit=max_throttle  LowerSaturationLimit=min_throttle
  Saturation : Saturate  UpperLimit=max_throttle_rate  LowerLimit=-max_throttle_rate
  Sum : Sum  Inputs=-+|  SaturateOnIntegerOverflow=on  InputSameDT=on  OutDataTypeStr=Inherit: Same as first input
  Throttle Time Constant : Gain  Gain=1/tau_throttle  SaturateOnIntegerOverflow=on  OutDataTypeStr=Inherit: Same as input  ParamDataTypeStr=Inherit: Same as input
  Angle : Outport
  wires:
  Command/1 -> Sum/2
  Integrator/1 -> Angle/1, Sum/1
  Sum/1 -> Throttle Time Constant/1
  Throttle Time Constant/1 -> Saturation/1
  Saturation/1 -> Integrator/1

== system platoon_project_string_stability3/2nd Vehicle/Vehicle Dynamics ==
  note: 타이어저항 F_road
  note: v
  note: v_dot
  note: 공기저항 F_air
  note: 구름저항 F_roll
  note: Initial Velocity = 21 [m/s]
  Tractive Force : Inport
  Aerodynamic Drag : Fcn  Expr=c_aero*u^2
  Divide by Mass : Gain  Gain=1/mass  Multiplication=Matrix(K*u)  SaturateOnIntegerOverflow=on  OutDataTypeStr=Inherit: Same as input  ParamDataTypeStr=Inherit: Same as input
  Integrator : Integrator  InitialCondition=x_dot_o  LimitOutput=on  LowerSaturationLimit=0
  Rolling Resistance : Constant  Value=F_roll
  Sum1 : Sum  Inputs=--+  SaturateOnIntegerOverflow=on  InputSameDT=on  OutDataTypeStr=Inherit: Same as first input
  Velocity : Outport
  Acceleration : Outport  Port=2
  wires:
  Tractive Force/1 -> Sum1/3
  Divide by Mass/1 -> Acceleration/1, Integrator/1
  Integrator/1 -> Velocity/1, Aerodynamic Drag/1
  Sum1/1 -> Divide by Mass/1
  Rolling Resistance/1 -> Sum1/2
  Aerodynamic Drag/1 -> Sum1/1

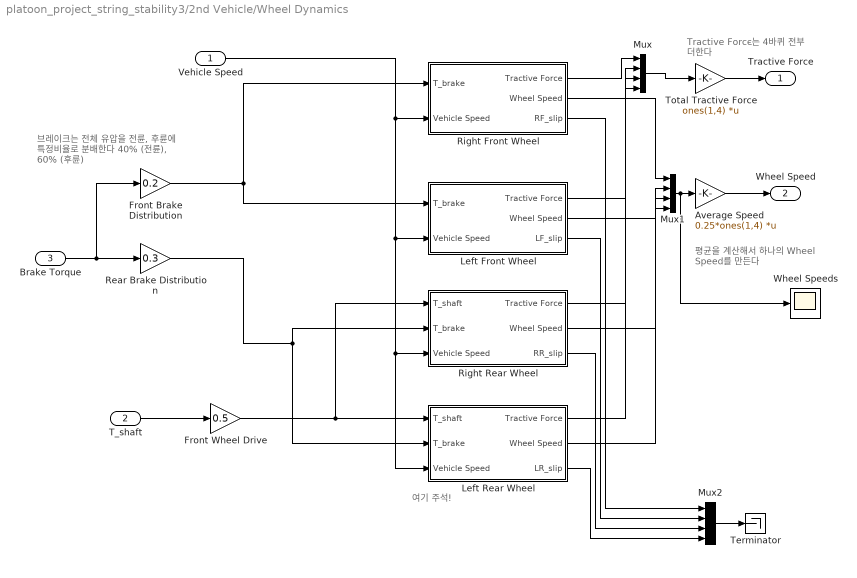
== system platoon_project_string_stability3/2nd Vehicle/Wheel Dynamics ==
  note: 여기 주석!
  note: Tractive Force는 4바퀴 전부 더한다
  note: 평균을 계산해서 하나의 Wheel Speed를 만든다
  note: 브레이크는 전체 유압을
      | 전륜, 후륜에 특정비율로 분배한다
      | 40% (전륜), 60% (후륜)
  Vehicle Speed : Inport
  T_shaft : Inport  Port=2
  Brake Torque : Inport  Port=3
  Average Speed : Gain  Gain=0.25*ones(1,4)  Multiplication=Matrix(K*u)  SaturateOnIntegerOverflow=on  OutDataTypeStr=Inherit: Same as input  ParamDataTypeStr=Inherit: Same as input
  Front Brake Distribution : Gain  Gain=0.2  SaturateOnIntegerOverflow=on  OutDataTypeStr=Inherit: Same as input  ParamDataTypeStr=Inherit: Same as input
  Front Wheel Drive : Gain  Gain=0.5  SaturateOnIntegerOverflow=on  OutDataTypeStr=Inherit: Same as input  ParamDataTypeStr=Inherit: Same as input
  Left Front Wheel : Subsystem
  Left Rear Wheel : Subsystem
  Mux : Mux
  Mux1 : Mux
  Mux2 : Mux
  Rear Brake Distribution : Gain  Gain=0.3  SaturateOnIntegerOverflow=on  OutDataTypeStr=Inherit: Same as input  ParamDataTypeStr=Inherit: Same as input
  Right Front Wheel : Subsystem
  Right Rear Wheel : Subsystem
  Terminator : Terminator
  Total Tractive Force : Gain  Gain=ones(1,4)  Multiplication=Matrix(K*u)  SaturateOnIntegerOverflow=on  OutDataTypeStr=Inherit: Same as input  ParamDataTypeStr=Inherit: Same as input
  Wheel Speeds : Scope
  Tractive Force : Outport
  Wheel Speed : Outport  Port=2
  wires:
  Total Tractive Force/1 -> Tractive Force/1
  Average Speed/1 -> Wheel Speed/1
  Mux/1 -> Total Tractive Force/1
  Vehicle Speed/1 -> Right Front Wheel/2(Vehicle Speed), Left Rear Wheel/3(Vehicle Speed), Right Rear Wheel/3(Vehicle Speed), Left Front Wheel/2(Vehicle Speed)
  Right Front Wheel/1(Tractive Force) -> Mux/1
  Left Front Wheel/1(Tractive Force) -> Mux/2
  Right Rear Wheel/1(Tractive Force) -> Mux/3
  Left Rear Wheel/1(Tractive Force) -> Mux/4
  Mux1/1 -> Average Speed/1, Wheel Speeds/1
  Right Front Wheel/2(Wheel Speed) -> Mux1/1
  Left Front Wheel/2(Wheel Speed) -> Mux1/2
  Right Rear Wheel/2(Wheel Speed) -> Mux1/3
  Left Rear Wheel/2(Wheel Speed) -> Mux1/4
  Right Front Wheel/3(RF_slip) -> Mux2/1
  Left Rear Wheel/3(LR_slip) -> Mux2/4
  Mux2/1 -> Terminator/1
  T_shaft/1 -> Front Wheel Drive/1
  Front Wheel Drive/1 -> Right Rear Wheel/1(T_shaft), Left Rear Wheel/1(T_shaft)
  Brake Torque/1 -> Rear Brake Distribution/1, Front Brake Distribution/1
  Left Front Wheel/3(LF_slip) -> Mux2/2
  Right Rear Wheel/3(RR_slip) -> Mux2/3
  Front Brake Distribution/1 -> Right Front Wheel/1(T_brake), Left Front Wheel/1(T_brake)
  Rear Brake Distribution/1 -> Left Rear Wheel/2(T_brake), Right Rear Wheel/2(T_brake)

== system platoon_project_string_stability3/3rd Vehicle/Brake Model ==
  note: Valve를 여닫는 시간에 따라
      | 필연적으로 발생하는 Time Delay
  note: brake는 1차 전달함수의 response를 보인다
  note: Wheel pressure
  note: Wheel Pressure가 브레이크 패드에 있는
      | Spring(k)보다 크게 걸렸을 때에만 브레이크가 작동하므로
      | Dead Zone이 발생한다
  Pmcc : Inport
  Brake Coefficient : Gain  Gain=KB  SaturateOnIntegerOverflow=on  OutDataTypeStr=Inherit: Same as input  ParamDataTypeStr=Inherit: Same as input
  Brake Dynamics : TransferFcn  Denominator=[tau_brake 1]
  Dead Zone : DeadZone  LowerValue=-P_po  UpperValue=P_po  SaturateOnIntegerOverflow=on
  Pure Time Delay : TransportDelay  DelayTime=delay_brake
  T_brake : Outport
  P_wheel : Outport  Port=2
  wires:
  Pure Time Delay/1 -> Brake Dynamics/1
  Pmcc/1 -> Pure Time Delay/1
  Brake Dynamics/1 -> Dead Zone/1, P_wheel/1  "P_wheel"
  Dead Zone/1 -> Brake Coefficient/1
  Brake Coefficient/1 -> T_brake/1

== system platoon_project_string_stability3/3rd Vehicle/Engine Model ==
  note: engine map이 저장되어있다
      | 2-D Lookup table
      |
      | input : Throttle angle, Engine speed
      | output : Engine torque
  Tractive Force : Inport
  Throttle Angle : Inport  Port=2
  Brake Torque : Inport  Port=3
  Gear Ratio : Inport  Port=4
  1/(I_e+4*I_w*R^2) : Fcn  Expr=u(1)/(I_e+4*I_wheel*u(2)^2)
  Integrator : Integrator  InitialCondition=we_o  LimitOutput=on  UpperSaturationLimit=[we_max]  LowerSaturationLimit=[we_min]
  Mux : Mux  Inputs=2
  Product : Product  SaturateOnIntegerOverflow=on  RndMeth=Zero  InputSameDT=on  OutDataTypeStr=Inherit: Same as first input
  Sum : Sum  Inputs=+|-  SaturateOnIntegerOverflow=on  InputSameDT=on  OutDataTypeStr=Inherit: Same as first input
  Sum1 : Sum  SaturateOnIntegerOverflow=on  InputSameDT=on  OutDataTypeStr=Inherit: Same as first input
  T_net : Lookup2D  RowIndex=alpha_table  ColumnIndex=we_table  Table=tnet_table  SaturateOnIntegerOverflow=on  InputSameDT=on
  wheel radius : Gain  Gain=h  Multiplication=Matrix(K*u)  SaturateOnIntegerOverflow=on  OutDataTypeStr=Inherit: Same as input  ParamDataTypeStr=Inherit: Same as input
  Engine Speed : Outport
  Engine Torque : Outport  Port=2
  wires:
  T_net/1 -> Sum/1, Engine Torque/1
  Mux/1 -> 1/(I_e+4*I_w*R^2)/1
  Sum/1 -> Mux/1
  Gear Ratio/1 -> Mux/2, Product/2
  Sum1/1 -> Product/1
  Product/1 -> Sum/2
  Brake Torque/1 -> Sum1/2
  wheel radius/1 -> Sum1/1
  Tractive Force/1 -> wheel radius/1
  1/(I_e+4*I_w*R^2)/1 -> Integrator/1  "w_dot"
  Integrator/1 -> T_net/2, Engine Speed/1  "w"
  Throttle Angle/1 -> T_net/1

== system platoon_project_string_stability3/3rd Vehicle/Gear Shift ==
  note: 현재 차량 속도 vs 기어변속 속도를 비교한다
      | [0; 1; 1] 같은 [1,n]행렬이 반환된다
  note: [1 1 1]인 [n,1] 행렬과
      | 반환행렬을 곱해서
      | 스칼라값(기어값)을 만든다
  Vehicle Speed : Inport
  Convert m/s to mph : Gain  Gain=3.6/1.6  SaturateOnIntegerOverflow=on  OutDataTypeStr=Inherit: Same as input  ParamDataTypeStr=Inherit: Same as input
  Direct Look-Up of Gear ratio : LookupNDDirect  NumberOfTableDimensions=1  Table=[0.3423,0.6378,1.0,1.4184]
  Get gear-1 : Gain  Gain=ones(1,3)  Multiplication=Matrix(K*u)  SaturateOnIntegerOverflow=on  OutDataTypeStr=Inherit: Same as input  ParamDataTypeStr=Inherit: Same as input
  Relational Operator : RelationalOperator  Operator=>  RndMeth=Nearest  InputSameDT=on
  Shift Speeds : Constant  Value=[15 32 67]
  Gear Ratio : Outport
  wires:
  Direct Look-Up of Gear ratio/1 -> Gear Ratio/1
  Vehicle Speed/1 -> Convert m/s to mph/1
  Get gear-1/1 -> Direct Look-Up of Gear ratio/1
  Convert m/s to mph/1 -> Relational Operator/1
  Relational Operator/1 -> Get gear-1/1
  Shift Speeds/1 -> Relational Operator/2

== system platoon_project_string_stability3/3rd Vehicle/Throttle Actuator ==
  Command : Inport
  Integrator : Integrator  InitialCondition=throttle_o  LimitOutput=on  UpperSaturationLimit=max_throttle  LowerSaturationLimit=min_throttle
  Saturation : Saturate  UpperLimit=max_throttle_rate  LowerLimit=-max_throttle_rate
  Sum : Sum  Inputs=-+|  SaturateOnIntegerOverflow=on  InputSameDT=on  OutDataTypeStr=Inherit: Same as first input
  Throttle Time Constant : Gain  Gain=1/tau_throttle  SaturateOnIntegerOverflow=on  OutDataTypeStr=Inherit: Same as input  ParamDataTypeStr=Inherit: Same as input
  Angle : Outport
  wires:
  Saturation/1 -> Integrator/1
  Throttle Time Constant/1 -> Saturation/1
  Sum/1 -> Throttle Time Constant/1
  Integrator/1 -> Sum/1, Angle/1
  Command/1 -> Sum/2

== system platoon_project_string_stability3/3rd Vehicle/Vehicle Dynamics ==
  note: 구름저항 F_roll
  note: 공기저항 F_air
  note: v_dot
  note: v
  note: 타이어저항 F_road
  note: Initial Velocity = 21 [m/s]
  Tractive Force : Inport
  Aerodynamic Drag : Fcn  Expr=c_aero*u^2
  Divide by Mass : Gain  Gain=1/mass  Multiplication=Matrix(K*u)  SaturateOnIntegerOverflow=on  OutDataTypeStr=Inherit: Same as input  ParamDataTypeStr=Inherit: Same as input
  Integrator : Integrator  InitialCondition=x_dot_o  LimitOutput=on  LowerSaturationLimit=0
  Rolling Resistance : Constant  Value=F_roll
  Sum1 : Sum  Inputs=--+  SaturateOnIntegerOverflow=on  InputSameDT=on  OutDataTypeStr=Inherit: Same as first input
  Velocity : Outport
  Acceleration : Outport  Port=2
  wires:
  Aerodynamic Drag/1 -> Sum1/1
  Rolling Resistance/1 -> Sum1/2
  Sum1/1 -> Divide by Mass/1
  Integrator/1 -> Aerodynamic Drag/1, Velocity/1
  Divide by Mass/1 -> Integrator/1, Acceleration/1
  Tractive Force/1 -> Sum1/3

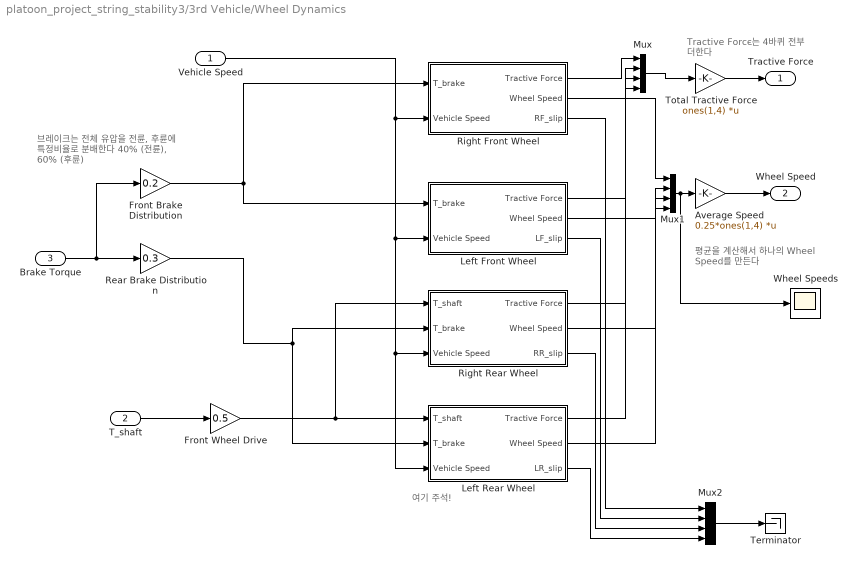
== system platoon_project_string_stability3/3rd Vehicle/Wheel Dynamics ==
  note: 브레이크는 전체 유압을
      | 전륜, 후륜에 특정비율로 분배한다
      | 40% (전륜), 60% (후륜)
  note: 평균을 계산해서 하나의 Wheel Speed를 만든다
  note: Tractive Force는 4바퀴 전부 더한다
  note: 여기 주석!
  Vehicle Speed : Inport
  T_shaft : Inport  Port=2
  Brake Torque : Inport  Port=3
  Average Speed : Gain  Gain=0.25*ones(1,4)  Multiplication=Matrix(K*u)  SaturateOnIntegerOverflow=on  OutDataTypeStr=Inherit: Same as input  ParamDataTypeStr=Inherit: Same as input
  Front Brake Distribution : Gain  Gain=0.2  SaturateOnIntegerOverflow=on  OutDataTypeStr=Inherit: Same as input  ParamDataTypeStr=Inherit: Same as input
  Front Wheel Drive : Gain  Gain=0.5  SaturateOnIntegerOverflow=on  OutDataTypeStr=Inherit: Same as input  ParamDataTypeStr=Inherit: Same as input
  Left Front Wheel : Subsystem
  Left Rear Wheel : Subsystem
  Mux : Mux
  Mux1 : Mux
  Mux2 : Mux
  Rear Brake Distribution : Gain  Gain=0.3  SaturateOnIntegerOverflow=on  OutDataTypeStr=Inherit: Same as input  ParamDataTypeStr=Inherit: Same as input
  Right Front Wheel : Subsystem
  Right Rear Wheel : Subsystem
  Terminator : Terminator
  Total Tractive Force : Gain  Gain=ones(1,4)  Multiplication=Matrix(K*u)  SaturateOnIntegerOverflow=on  OutDataTypeStr=Inherit: Same as input  ParamDataTypeStr=Inherit: Same as input
  Wheel Speeds : Scope
  Tractive Force : Outport
  Wheel Speed : Outport  Port=2
  wires:
  Rear Brake Distribution/1 -> Right Rear Wheel/2(T_brake), Left Rear Wheel/2(T_brake)
  Front Brake Distribution/1 -> Left Front Wheel/1(T_brake), Right Front Wheel/1(T_brake)
  Right Rear Wheel/3(RR_slip) -> Mux2/3
  Left Front Wheel/3(LF_slip) -> Mux2/2
  Brake Torque/1 -> Front Brake Distribution/1, Rear Brake Distribution/1
  Front Wheel Drive/1 -> Left Rear Wheel/1(T_shaft), Right Rear Wheel/1(T_shaft)
  T_shaft/1 -> Front Wheel Drive/1
  Mux2/1 -> Terminator/1
  Left Rear Wheel/3(LR_slip) -> Mux2/4
  Right Front Wheel/3(RF_slip) -> Mux2/1
  Left Rear Wheel/2(Wheel Speed) -> Mux1/4
  Right Rear Wheel/2(Wheel Speed) -> Mux1/3
  Left Front Wheel/2(Wheel Speed) -> Mux1/2
  Right Front Wheel/2(Wheel Speed) -> Mux1/1
  Mux1/1 -> Wheel Speeds/1, Average Speed/1
  Left Rear Wheel/1(Tractive Force) -> Mux/4
  Right Rear Wheel/1(Tractive Force) -> Mux/3
  Left Front Wheel/1(Tractive Force) -> Mux/2
  Right Front Wheel/1(Tractive Force) -> Mux/1
  Vehicle Speed/1 -> Left Front Wheel/2(Vehicle Speed), Right Rear Wheel/3(Vehicle Speed), Left Rear Wheel/3(Vehicle Speed), Right Front Wheel/2(Vehicle Speed)
  Mux/1 -> Total Tractive Force/1
  Average Speed/1 -> Wheel Speed/1
  Total Tractive Force/1 -> Tractive Force/1

== system platoon_project_string_stability3/4th Vehicle/Brake Model ==
  note: Wheel Pressure가 브레이크 패드에 있는
      | Spring(k)보다 크게 걸렸을 때에만 브레이크가 작동하므로
      | Dead Zone이 발생한다
  note: Wheel pressure
  note: brake는 1차 전달함수의 response를 보인다
  note: Valve를 여닫는 시간에 따라
      | 필연적으로 발생하는 Time Delay
  Pmcc : Inport
  Brake Coefficient : Gain  Gain=KB  SaturateOnIntegerOverflow=on  OutDataTypeStr=Inherit: Same as input  ParamDataTypeStr=Inherit: Same as input
  Brake Dynamics : TransferFcn  Denominator=[tau_brake 1]
  Dead Zone : DeadZone  LowerValue=-P_po  UpperValue=P_po  SaturateOnIntegerOverflow=on
  Pure Time Delay : TransportDelay  DelayTime=delay_brake
  T_brake : Outport
  P_wheel : Outport  Port=2
  wires:
  Brake Coefficient/1 -> T_brake/1
  Dead Zone/1 -> Brake Coefficient/1
  Brake Dynamics/1 -> P_wheel/1, Dead Zone/1  "P_wheel"
  Pmcc/1 -> Pure Time Delay/1
  Pure Time Delay/1 -> Brake Dynamics/1

== system platoon_project_string_stability3/4th Vehicle/Engine Model ==
  note: engine map이 저장되어있다
      | 2-D Lookup table
      |
      | input : Throttle angle, Engine speed
      | output : Engine torque
  Tractive Force : Inport
  Throttle Angle : Inport  Port=2
  Brake Torque : Inport  Port=3
  Gear Ratio : Inport  Port=4
  1/(I_e+4*I_w*R^2) : Fcn  Expr=u(1)/(I_e+4*I_wheel*u(2)^2)
  Integrator : Integrator  InitialCondition=we_o  LimitOutput=on  UpperSaturationLimit=[we_max]  LowerSaturationLimit=[we_min]
  Mux : Mux  Inputs=2
  Product : Product  SaturateOnIntegerOverflow=on  RndMeth=Zero  InputSameDT=on  OutDataTypeStr=Inherit: Same as first input
  Sum : Sum  Inputs=+|-  SaturateOnIntegerOverflow=on  InputSameDT=on  OutDataTypeStr=Inherit: Same as first input
  Sum1 : Sum  SaturateOnIntegerOverflow=on  InputSameDT=on  OutDataTypeStr=Inherit: Same as first input
  T_net : Lookup2D  RowIndex=alpha_table  ColumnIndex=we_table  Table=tnet_table  SaturateOnIntegerOverflow=on  InputSameDT=on
  wheel radius : Gain  Gain=h  Multiplication=Matrix(K*u)  SaturateOnIntegerOverflow=on  OutDataTypeStr=Inherit: Same as input  ParamDataTypeStr=Inherit: Same as input
  Engine Speed : Outport
  Engine Torque : Outport  Port=2
  wires:
  Throttle Angle/1 -> T_net/1
  Integrator/1 -> Engine Speed/1, T_net/2  "w"
  1/(I_e+4*I_w*R^2)/1 -> Integrator/1  "w_dot"
  Tractive Force/1 -> wheel radius/1
  wheel radius/1 -> Sum1/1
  Brake Torque/1 -> Sum1/2
  Product/1 -> Sum/2
  Sum1/1 -> Product/1
  Gear Ratio/1 -> Product/2, Mux/2
  Sum/1 -> Mux/1
  Mux/1 -> 1/(I_e+4*I_w*R^2)/1
  T_net/1 -> Engine Torque/1, Sum/1

== system platoon_project_string_stability3/4th Vehicle/Gear Shift ==
  note: [1 1 1]인 [n,1] 행렬과
      | 반환행렬을 곱해서
      | 스칼라값(기어값)을 만든다
  note: 현재 차량 속도 vs 기어변속 속도를 비교한다
      | [0; 1; 1] 같은 [1,n]행렬이 반환된다
  Vehicle Speed : Inport
  Convert m/s to mph : Gain  Gain=3.6/1.6  SaturateOnIntegerOverflow=on  OutDataTypeStr=Inherit: Same as input  ParamDataTypeStr=Inherit: Same as input
  Direct Look-Up of Gear ratio : LookupNDDirect  NumberOfTableDimensions=1  Table=[0.3423,0.6378,1.0,1.4184]
  Get gear-1 : Gain  Gain=ones(1,3)  Multiplication=Matrix(K*u)  SaturateOnIntegerOverflow=on  OutDataTypeStr=Inherit: Same as input  ParamDataTypeStr=Inherit: Same as input
  Relational Operator : RelationalOperator  Operator=>  RndMeth=Nearest  InputSameDT=on
  Shift Speeds : Constant  Value=[15 32 67]
  Gear Ratio : Outport
  wires:
  Shift Speeds/1 -> Relational Operator/2
  Relational Operator/1 -> Get gear-1/1
  Convert m/s to mph/1 -> Relational Operator/1
  Get gear-1/1 -> Direct Look-Up of Gear ratio/1
  Vehicle Speed/1 -> Convert m/s to mph/1
  Direct Look-Up of Gear ratio/1 -> Gear Ratio/1

== system platoon_project_string_stability3/4th Vehicle/Throttle Actuator ==
  Command : Inport
  Integrator : Integrator  InitialCondition=throttle_o  LimitOutput=on  UpperSaturationLimit=max_throttle  LowerSaturationLimit=min_throttle
  Saturation : Saturate  UpperLimit=max_throttle_rate  LowerLimit=-max_throttle_rate
  Sum : Sum  Inputs=-+|  SaturateOnIntegerOverflow=on  InputSameDT=on  OutDataTypeStr=Inherit: Same as first input
  Throttle Time Constant : Gain  Gain=1/tau_throttle  SaturateOnIntegerOverflow=on  OutDataTypeStr=Inherit: Same as input  ParamDataTypeStr=Inherit: Same as input
  Angle : Outport
  wires:
  Command/1 -> Sum/2
  Integrator/1 -> Angle/1, Sum/1
  Sum/1 -> Throttle Time Constant/1
  Throttle Time Constant/1 -> Saturation/1
  Saturation/1 -> Integrator/1

== system platoon_project_string_stability3/4th Vehicle/Vehicle Dynamics ==
  note: 타이어저항 F_road
  note: v
  note: v_dot
  note: 공기저항 F_air
  note: 구름저항 F_roll
  note: Initial Velocity = 21 [m/s]
  Tractive Force : Inport
  Aerodynamic Drag : Fcn  Expr=c_aero*u^2
  Divide by Mass : Gain  Gain=1/mass  Multiplication=Matrix(K*u)  SaturateOnIntegerOverflow=on  OutDataTypeStr=Inherit: Same as input  ParamDataTypeStr=Inherit: Same as input
  Integrator : Integrator  InitialCondition=x_dot_o  LimitOutput=on  LowerSaturationLimit=0
  Rolling Resistance : Constant  Value=F_roll
  Sum1 : Sum  Inputs=--+  SaturateOnIntegerOverflow=on  InputSameDT=on  OutDataTypeStr=Inherit: Same as first input
  Velocity : Outport
  Acceleration : Outport  Port=2
  wires:
  Tractive Force/1 -> Sum1/3
  Divide by Mass/1 -> Acceleration/1, Integrator/1
  Integrator/1 -> Velocity/1, Aerodynamic Drag/1
  Sum1/1 -> Divide by Mass/1
  Rolling Resistance/1 -> Sum1/2
  Aerodynamic Drag/1 -> Sum1/1
